simulink model "M_DCMotor_MPC"  (R2019a)
settings: Solver=FixedStepDiscrete  StartTime=0.0  StopTime=18.0  FixedStep=0.0001  RelTol=1e-3
values from neighbouring files (symbols this model uses):
  J = 0.02    [Startfile_M_DCmotor_MPC.m]
  Kemf = 0.1    [Startfile_M_DCmotor_MPC.m]
  Kf = 0.2    [Startfile_M_DCmotor_MPC.m]
  Km = 0.1    [Startfile_M_DCmotor_MPC.m]
  L = 0.5    [Startfile_M_DCmotor_MPC.m]
  Q0_DC_MPC = [0.01 40000 40000 10]    [Startfile_M_DCmotor_MPC.m]
  R = 2    [Startfile_M_DCmotor_MPC.m]
  R0_DC_MPC = 0.01    [Startfile_M_DCmotor_MPC.m]
  SampleTime = 0.0001    [Startfile_M_DCmotor_MPC.m]
undefined symbols (not defined in the file or in its folder): serial
libraries: powerlib x24, instrumentlib x3
settings Model: Creator=simon  LastModifiedBy=simon
settings OptimizationCC: DefaultParameterBehavior=Inlined  EnhancedBackFolding=on  PassReuseOutputArgsAs=Individual arguments  OptimizeBlockOrder=speed  DifferentSizesBufferReuse=on
settings DebuggingCC: ParameterTunabilityLossMsg=error
settings HardwareCC: ProdBitPerPointer=32  ProdBitPerSizeT=32  ProdBitPerPtrDiffT=32  ProdLargestAtomicInteger=Long  ProdLargestAtomicFloat=Double  ProdWordSize=32  ProdHWDeviceType=ARM Compatible->ARM Cortex
settings SFSimCC: MATLABDynamicMemAlloc=off
settings RTWCC: SystemTargetFile=ert.tlc  TemplateMakefile=ert_default_tmf  GenerateReport=on  RTWUseSimCustomCode=on  IncludeHyperlinkInReport=on  LaunchReport=on  GenerateTraceInfo=on  GenerateTraceReport=on  GenerateTraceReportSl=on  GenerateTraceReportSf=on  GenerateTraceReportEml=on  GenerateCodeMetricsReport=on
settings CodeAppCC: ForceParamTrailComments=on  IgnoreCustomStorageClasses=off  OperatorAnnotations=on  SimulinkDataObjDesc=on  SFDataObjDesc=on  InsertBlockDesc=on
settings ERTTargetCC: TargetLangStandard=C99 (ISO)  GenerateSampleERTMain=on  InlinedParameterPlacement=NonHierarchical  ERTCustomFileTemplate=example_file_process.tlc  GlobalDataDefinition=InSeparateSourceFile  GlobalDataReference=InSeparateHeaderFile  ERTFilePackagingFormat=CompactWithDataFile

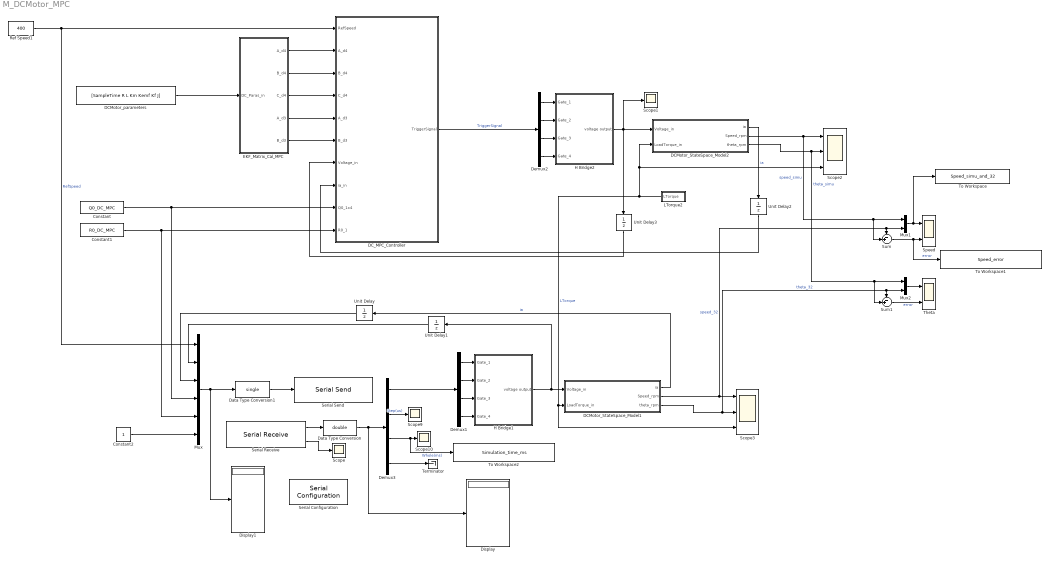
== system M_DCMotor_MPC ==
  Constant : Constant  Value=Q0_DC_MPC
  Constant1 : Constant  Value=R0_DC_MPC
  Constant2 : Constant
  DCMotor_StateSpace_Model1 : Subsystem
  DCMotor_StateSpace_Model2 : Subsystem
  DCMotor_parameters : Constant  Value=[SampleTime R L Km Kemf Kf J]
  DC_MPC_Controller : Subsystem
  Data Type Conversion : DataTypeConversion  OutDataTypeStr=double
  Data Type Conversion1 : DataTypeConversion  OutDataTypeStr=single
  Demux1 : Demux
  Demux2 : Demux
  Demux3 : Demux  Outputs=[4 1 1 3]
  Display : Display
  Display1 : Display
  EKF_Matrix_Cal_MPC : MATLAB Function  TreatAsAtomicUnit=on
  H Bridge1 : Subsystem
  H Bridge2 : Subsystem
  LTorque2 : Subsystem
  Mux : Mux  Inputs=6
  Mux1 : Mux  Inputs=2
  Mux2 : Mux  Inputs=2
  Ref Speed1 : Constant  Value=400
  Scope{,1,9..10} (4 alike) : Scope
  Scope2 : Scope  NumInputPorts=3
  Scope3 : Scope  NumInputPorts=3
  Serial Configuration : instrumentlib/Serial Configuration  Priority=-200000  ComPortMenu=<Please select a port...>  ComPort=/dev/cu.usbmodem141303  ObjConstructor=serial('/dev/cu.usbmodem141303');  BaudRate=921600  DataBits=8  Parity=none  StopBits=1  FlowControl=none  Timeout=10  ByteOrder=LittleEndian
  Serial Receive : instrumentlib/Serial Receive  ComPortMenu=<Please select a port...>  ComPort=/dev/cu.usbmodem141303  ObjConstructor=serial('/dev/cu.usbmodem141303');  Terminator=<none>  DataSize="[1  9]"  DataType=single  EnableBlockingMode=off  ActionDataUnavailable=Output last received value  CustomValue=0  SampleTime=SampleTime
  Serial Send : instrumentlib/Serial Send  ComPortMenu=<Please select a port...>  ComPort=/dev/cu.usbmodem141303  ObjConstructor=serial('/dev/cu.usbmodem141303');  Terminator=<none>  EnableBlockingMode=off
  Speed : Scope  NumInputPorts=2
  Sum : Sum  Inputs=-+|
  Sum1 : Sum  Inputs=-+|
  Terminator : Terminator
  Theta : Scope  NumInputPorts=2
  To Workspace : ToWorkspace  VariableName=Speed_simu_and_32  SampleTime=-1
      settings: Save2DSignal=2-D array (concatenate along first dimension)
  To Workspace1 : ToWorkspace  VariableName=Speed_error  SampleTime=-1
      settings: Save2DSignal=2-D array (concatenate along first dimension)
  To Workspace2 : ToWorkspace  VariableName=Simulation_time_ms  SampleTime=-1
      settings: Save2DSignal=2-D array (concatenate along first dimension)
  Unit Delay{,1..3} (4 alike) : UnitDelay  SampleTime=-1  HasFrameUpgradeWarning=on
  wires:
  DCMotor_parameters/1 -> EKF_Matrix_Cal_MPC/1(DC_Paras_in)
  EKF_Matrix_Cal_MPC/1(A_d4) -> DC_MPC_Controller/2(A_d4)
  EKF_Matrix_Cal_MPC/2(B_d4) -> DC_MPC_Controller/3(B_d4)
  EKF_Matrix_Cal_MPC/3(C_d4) -> DC_MPC_Controller/4(C_d4)
  Constant/1 -> Mux/4, DC_MPC_Controller/9(Q0_1x4)
  Constant1/1 -> Mux/5, DC_MPC_Controller/10(R0_1)
  LTorque2/1(LTorque) -> Scope3/3, DCMotor_StateSpace_Model1/2(LoadTorque_in), DCMotor_StateSpace_Model2/2(LoadTorque_in), Scope2/3  "LTorque"
  Demux2/1 -> H Bridge2/1(Gate_1)
  Demux2/4 -> H Bridge2/4(Gate_4)
  Demux2/3 -> H Bridge2/3(Gate_3)
  H Bridge2/1(voltage output) -> Unit Delay3/1, DCMotor_StateSpace_Model2/1(Voltage_in), Scope1/1
  DC_MPC_Controller/1(TriggerSignal) -> Demux2/1  "TriggerSignal"
  Demux2/2 -> H Bridge2/2(Gate_2)
  DCMotor_StateSpace_Model2/1(ia) -> Unit Delay2/1  "ia"
  DCMotor_StateSpace_Model2/2(Speed_rpm) -> Sum/2, Mux1/1, Scope2/1  "speed_simu"
  DCMotor_StateSpace_Model2/3(theta_rpm) -> Sum1/2, Mux2/1, Scope2/2  "theta_simu"
  Ref Speed1/1 -> Mux/1, DC_MPC_Controller/1(RefSpeed)  "RefSpeed"
  EKF_Matrix_Cal_MPC/4(A_d3) -> DC_MPC_Controller/5(A_d3)
  EKF_Matrix_Cal_MPC/5(B_d3) -> DC_MPC_Controller/6(B_d3)
  Demux3/1 -> Demux1/1
  Demux3/2 -> Scope9/1  "Step(us)"
  Data Type Conversion/1 -> Display/1, Demux3/1
  Demux1/4 -> H Bridge1/4(Gate_4)
  Demux3/3 -> To Workspace2/1, Scope10/1  "Whole(ms)"
  Demux1/2 -> H Bridge1/2(Gate_2)
  Demux1/3 -> H Bridge1/3(Gate_3)
  Mux/1 -> Display1/1, Data Type Conversion1/1
  Demux1/1 -> H Bridge1/1(Gate_1)
  Data Type Conversion1/1 -> Serial Send/1
  Serial Receive/1 -> Data Type Conversion/1
  DCMotor_StateSpace_Model1/3(theta_rpm) -> Mux2/2, Sum1/1, Scope3/2  "theta_32"
  DCMotor_StateSpace_Model1/2(Speed_rpm) -> Sum/1, Mux1/2, Scope3/1  "speed_32"
  H Bridge1/1(voltage output) -> Unit Delay1/1, DCMotor_StateSpace_Model1/1(Voltage_in)
  DCMotor_StateSpace_Model1/1(ia) -> Unit Delay/1  "ia"
  Unit Delay2/1 -> DC_MPC_Controller/8(ia_in)
  Unit Delay3/1 -> DC_MPC_Controller/7(Voltage_in)
  Unit Delay/1 -> Mux/3
  Unit Delay1/1 -> Mux/2
  Demux3/4 -> Terminator/1
  Constant2/1 -> Mux/6
  Mux1/1 -> To Workspace/1, Speed/1
  Sum/1 -> To Workspace1/1, Speed/2  "error"
  Mux2/1 -> Theta/1
  Sum1/1 -> Theta/2  "error"
  Serial Receive/2 -> Scope/1

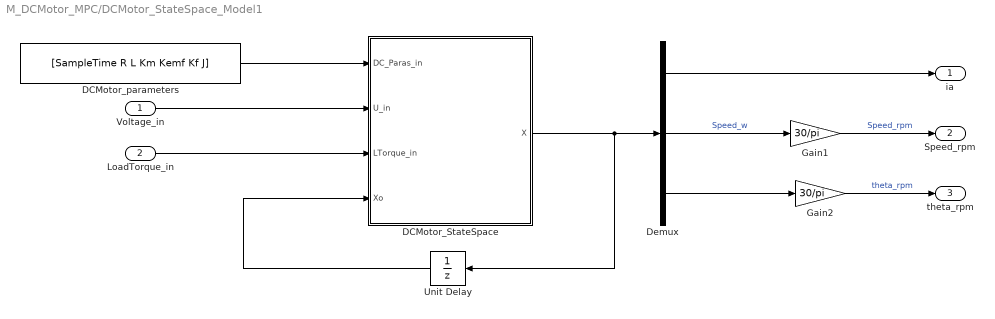
== system M_DCMotor_MPC/DCMotor_StateSpace_Model1 ==
  Voltage_in : Inport
  LoadTorque_in : Inport  Port=2
  DCMotor_StateSpace : MATLAB Function  TreatAsAtomicUnit=on
  DCMotor_parameters : Constant  Value=[SampleTime R L Km Kemf Kf J]
  Demux : Demux  Outputs=3
  Gain1 : Gain  Gain=30/pi
  Gain2 : Gain  Gain=30/pi
  Unit Delay : UnitDelay  SampleTime=-1  HasFrameUpgradeWarning=on
  ia : Outport
  Speed_rpm : Outport  Port=2
  theta_rpm : Outport  Port=3
  wires:
  Gain2/1 -> theta_rpm/1  "theta_rpm"
  Demux/3 -> Gain2/1
  Demux/1 -> ia/1
  Gain1/1 -> Speed_rpm/1  "Speed_rpm"
  Demux/2 -> Gain1/1  "Speed_w"
  DCMotor_StateSpace/1(X) -> Demux/1, Unit Delay/1
  DCMotor_parameters/1 -> DCMotor_StateSpace/1(DC_Paras_in)
  LoadTorque_in/1 -> DCMotor_StateSpace/3(LTorque_in)
  Unit Delay/1 -> DCMotor_StateSpace/4(Xo)
  Voltage_in/1 -> DCMotor_StateSpace/2(U_in)

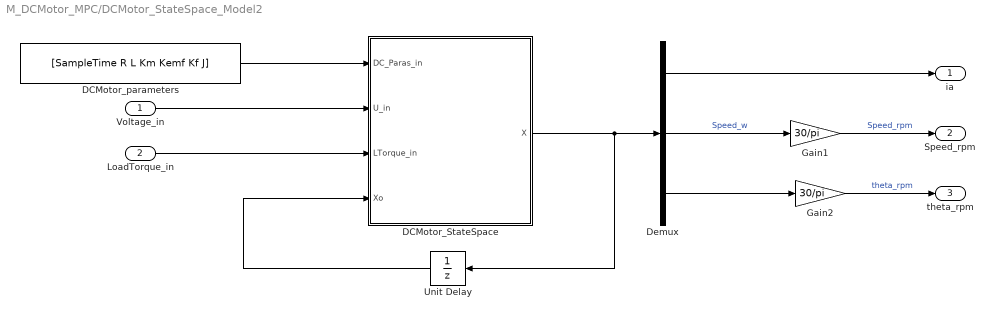
== system M_DCMotor_MPC/DCMotor_StateSpace_Model2 ==
  Voltage_in : Inport
  LoadTorque_in : Inport  Port=2
  DCMotor_StateSpace : MATLAB Function  TreatAsAtomicUnit=on
  DCMotor_parameters : Constant  Value=[SampleTime R L Km Kemf Kf J]
  Demux : Demux  Outputs=3
  Gain1 : Gain  Gain=30/pi
  Gain2 : Gain  Gain=30/pi
  Unit Delay : UnitDelay  SampleTime=-1  HasFrameUpgradeWarning=on
  ia : Outport
  Speed_rpm : Outport  Port=2
  theta_rpm : Outport  Port=3
  wires:
  Voltage_in/1 -> DCMotor_StateSpace/2(U_in)
  Unit Delay/1 -> DCMotor_StateSpace/4(Xo)
  LoadTorque_in/1 -> DCMotor_StateSpace/3(LTorque_in)
  DCMotor_parameters/1 -> DCMotor_StateSpace/1(DC_Paras_in)
  DCMotor_StateSpace/1(X) -> Unit Delay/1, Demux/1
  Demux/2 -> Gain1/1  "Speed_w"
  Gain1/1 -> Speed_rpm/1  "Speed_rpm"
  Demux/1 -> ia/1
  Demux/3 -> Gain2/1
  Gain2/1 -> theta_rpm/1  "theta_rpm"

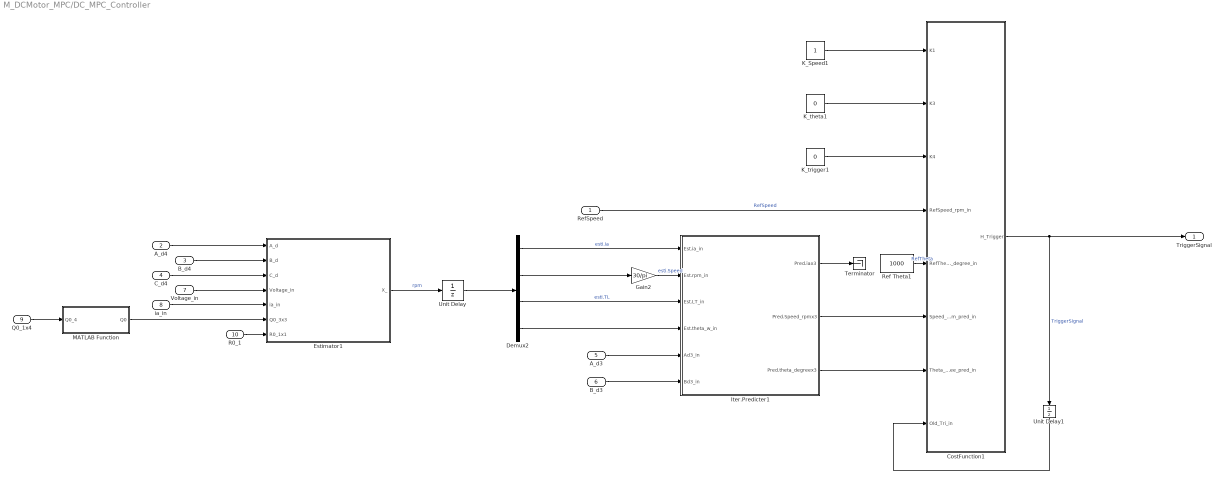
== system M_DCMotor_MPC/DC_MPC_Controller ==
  RefSpeed : Inport
  A_d4 : Inport  Port=2
  B_d4 : Inport  Port=3
  C_d4 : Inport  Port=4
  A_d3 : Inport  Port=5
  B_d3 : Inport  Port=6
  Voltage_in : Inport  Port=7
  ia_in : Inport  Port=8
  Q0_1x4 : Inport  Port=9
  R0_1 : Inport  Port=10
  CostFunction1 : MATLAB Function  TreatAsAtomicUnit=on
  Demux2 : Demux
  Estimator1 : Subsystem
  Gain2 : Gain  Gain=30/pi
  Iter.Predicter1 : Subsystem
  K_Speed1 : Constant
  K_theta1 : Constant  Value=0
  K_trigger1 : Constant  Value=0
  MATLAB Function : MATLAB Function  TreatAsAtomicUnit=on
  Ref Theta1 : Constant  Value=1000
  Terminator : Terminator
  Unit Delay : UnitDelay  SampleTime=-1  HasFrameUpgradeWarning=on
  Unit Delay1 : UnitDelay  SampleTime=-1  HasFrameUpgradeWarning=on
  TriggerSignal : Outport
  wires:
  K_theta1/1 -> CostFunction1/2(K3)
  ia_in/1 -> Estimator1/5(ia_in)
  Demux2/2 -> Gain2/1
  Ref Theta1/1 -> CostFunction1/5(RefTheta_degree_in)  "RefTheta"
  MATLAB Function/1(Q0) -> Estimator1/6(Q0_3x3)
  K_Speed1/1 -> CostFunction1/1(K1)
  R0_1/1 -> Estimator1/7(R0_1x1)
  RefSpeed/1 -> CostFunction1/4(RefSpeed_rpm_in)  "RefSpeed"
  A_d4/1 -> Estimator1/1(A_d)
  Unit Delay1/1 -> CostFunction1/8(Old_Tri_in)
  CostFunction1/1(H_Trigger) -> Unit Delay1/1, TriggerSignal/1  "TriggerSignal"
  Estimator1/1(X_) -> Unit Delay/1  "rpm"
  C_d4/1 -> Estimator1/3(C_d)
  Voltage_in/1 -> Estimator1/4(Voltage_in)
  Q0_1x4/1 -> MATLAB Function/1(Q0_4)
  B_d4/1 -> Estimator1/2(B_d)
  K_trigger1/1 -> CostFunction1/3(K4)
  Gain2/1 -> Iter.Predicter1/2(Est.rpm_in)  "esti.Speed"
  Demux2/3 -> Iter.Predicter1/3(Est.LT_in)  "esti.TL"
  Demux2/1 -> Iter.Predicter1/1(Est.ia_in)  "esti.ia"
  Iter.Predicter1/1(Pred.iax3) -> Terminator/1
  Demux2/4 -> Iter.Predicter1/4(Est.theta_w_in)
  A_d3/1 -> Iter.Predicter1/5(Ad3_in)
  B_d3/1 -> Iter.Predicter1/6(Bd3_in)
  Iter.Predicter1/2(Pred.Speed_rpmx3) -> CostFunction1/6(Speed_rpm_pred_in)
  Iter.Predicter1/3(Pred.theta_degreex3) -> CostFunction1/7(Theta_degree_pred_in)
  Unit Delay/1 -> Demux2/1

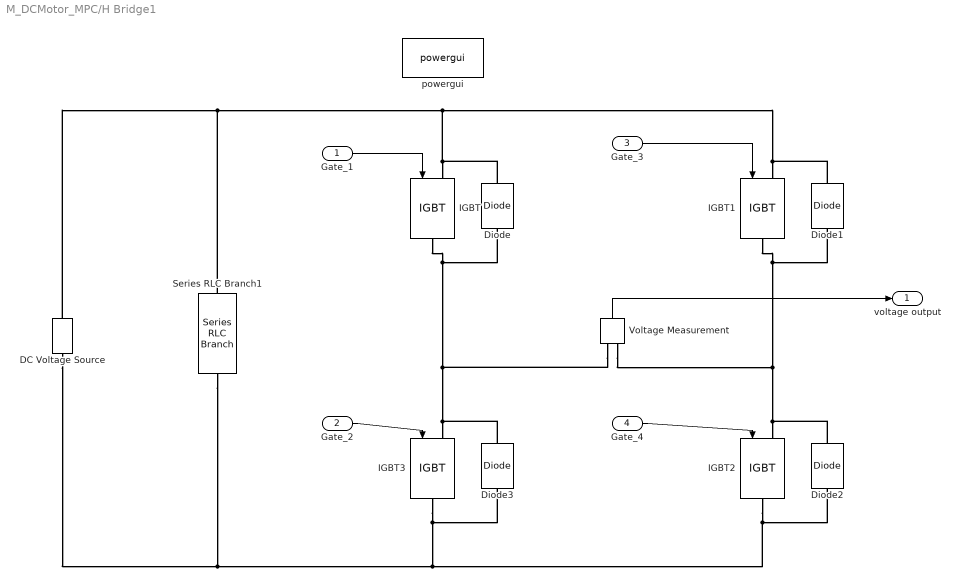
== system M_DCMotor_MPC/H Bridge1 ==
  Gate_1 : Inport
  Gate_2 : Inport  Port=2
  Gate_3 : Inport  Port=3
  Gate_4 : Inport  Port=4
  DC Voltage Source : powerlib/Electrical Sources/DC Voltage Source  Amplitude=400  Measurements=None
      settings: SourceProductName=Simscape Electrical
  Diode{,1..3} (4 alike) : powerlib/Power Electronics/Diode  Ron=0.001  Lon=0  Vf=0.8  IC=0  UseSnubber=0  Rs=500  Cs=250e-9  Measurements=off
      settings: SourceProductName=Simscape Electrical
  IGBT{,1..3} (4 alike) : powerlib/Power Electronics/IGBT  Ron=0.001  Lon=0  Vf=1  Tf=1e-6  Tt=2e-6  IC=0  Rs=1e5  Cs=inf  Measurements=off
      settings: SourceProductName=Simscape Electrical
  Series RLC Branch1 : powerlib/Elements/Series RLC Branch  LConnTagsString=__new0  RConnTagsString=__new0  BranchType=RC  Resistance=0.01  Inductance=1e-3  SetiL0=off  InitialCurrent=0  Capacitance=50e-6  Setx0=off  InitialVoltage=0  Measurements=None
      settings: SourceProductName=Simscape Electrical
  Voltage Measurement : powerlib/Measurements/Voltage Measurement  PhasorSimulation=off  OutputType=Complex  PSBequivalent=0
      settings: SourceProductName=Simscape Electrical
  powergui : powerlib/powergui  Priority=1  SimulationMode=Discrete  SampleTime=0.0001  frequency=60  Iterations=50  frequencyindice=0  Pbase=100e6  ErrMax=1e-4  UnitsV=kV  UnitsW=MW  buscounter=0  FunctionMessages=off  echomessages=off  EnableUseOfTLC=off  CurrentSourceSwitches=off  DisableSnubberDevices=off  DisableRonSwitches=off  DisableVfSwitches=off  DisplayEquations=off  AutomaticDiscreteSolvers=off  SolverType=Tustin/Backward Euler (TBE)  Interpol=off  ExternalGateDelay=off  methode=off  Ts=100  x0status=blocks  SPID=on  SwTol=0  HookPort=off  NonlinearTolerance=0  nMaxIteration=15  ContinueOnMaxIteration=off  RestoreLinks=warning  ResistiveCurrentMeasurement=off  Frange=[0:2:500]  Ylog=off  Xlog=on  ShowGrid=off  save=off  variable=ZData  structure=0  ZoomFFT=off  StartTime=0.0  cycles=1  DisplayStyle=1  fundamental=60  FreqAxis=off  MaxFrequency=1000  frequencyindicesteady=1  RmsSteady=1  display=off
      settings: SourceProductName=Simscape Electrical
  voltage output : Outport
  wires:
  Gate_1/1 -> IGBT/1
  Voltage Measurement/1 -> voltage output/1
  Gate_2/1 -> IGBT3/1
  Gate_3/1 -> IGBT1/1
  Gate_4/1 -> IGBT2/1
  connections:
  IGBT/RConn1 -- Voltage Measurement/LConn1 -- IGBT3/LConn1 -- Diode3/RConn1 -- Diode/LConn1
  Diode/RConn1 -- Series RLC Branch1/LConn1 -- DC Voltage Source/RConn1 -- IGBT1/LConn1 -- Diode1/RConn1 -- IGBT/LConn1
  IGBT1/RConn1 -- Voltage Measurement/LConn2 -- IGBT2/LConn1 -- Diode2/RConn1 -- Diode1/LConn1
  IGBT3/RConn1 -- DC Voltage Source/LConn1 -- Series RLC Branch1/RConn1 -- IGBT2/RConn1 -- Diode2/LConn1 -- Diode3/LConn1

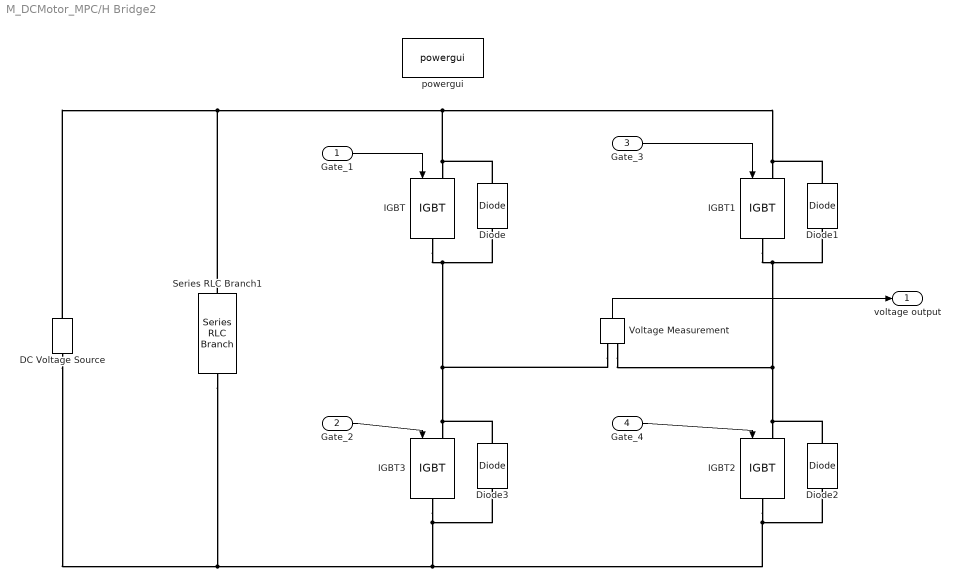
== system M_DCMotor_MPC/H Bridge2 ==
  Gate_1 : Inport
  Gate_2 : Inport  Port=2
  Gate_3 : Inport  Port=3
  Gate_4 : Inport  Port=4
  DC Voltage Source : powerlib/Electrical Sources/DC Voltage Source  Amplitude=400  Measurements=None
      settings: SourceProductName=Simscape Electrical
  Diode{,1..3} (4 alike) : powerlib/Power Electronics/Diode  Ron=0.001  Lon=0  Vf=0.8  IC=0  UseSnubber=0  Rs=500  Cs=250e-9  Measurements=off
      settings: SourceProductName=Simscape Electrical
  IGBT{,1..3} (4 alike) : powerlib/Power Electronics/IGBT  Ron=0.001  Lon=0  Vf=1  Tf=1e-6  Tt=2e-6  IC=0  Rs=1e5  Cs=inf  Measurements=off
      settings: SourceProductName=Simscape Electrical
  Series RLC Branch1 : powerlib/Elements/Series RLC Branch  LConnTagsString=__new0  RConnTagsString=__new0  BranchType=RC  Resistance=0.01  Inductance=1e-3  SetiL0=off  InitialCurrent=0  Capacitance=50e-6  Setx0=off  InitialVoltage=0  Measurements=None
      settings: SourceProductName=Simscape Electrical
  Voltage Measurement : powerlib/Measurements/Voltage Measurement  PhasorSimulation=off  OutputType=Complex  PSBequivalent=0
      settings: SourceProductName=Simscape Electrical
  powergui : powerlib/powergui  Priority=1  SimulationMode=Discrete  SampleTime=0.0001  frequency=60  Iterations=50  frequencyindice=0  Pbase=100e6  ErrMax=1e-4  UnitsV=kV  UnitsW=MW  buscounter=0  FunctionMessages=off  echomessages=off  EnableUseOfTLC=off  CurrentSourceSwitches=off  DisableSnubberDevices=off  DisableRonSwitches=off  DisableVfSwitches=off  DisplayEquations=off  AutomaticDiscreteSolvers=off  SolverType=Tustin/Backward Euler (TBE)  Interpol=off  ExternalGateDelay=off  methode=off  Ts=100  x0status=blocks  SPID=on  SwTol=0  HookPort=off  NonlinearTolerance=0  nMaxIteration=15  ContinueOnMaxIteration=off  RestoreLinks=warning  ResistiveCurrentMeasurement=off  Frange=[0:2:500]  Ylog=off  Xlog=on  ShowGrid=off  save=off  variable=ZData  structure=0  ZoomFFT=off  StartTime=0.0  cycles=1  DisplayStyle=1  fundamental=60  FreqAxis=off  MaxFrequency=1000  frequencyindicesteady=1  RmsSteady=1  display=off
      settings: SourceProductName=Simscape Electrical
  voltage output : Outport
  wires:
  Gate_1/1 -> IGBT/1
  Voltage Measurement/1 -> voltage output/1
  Gate_2/1 -> IGBT3/1
  Gate_3/1 -> IGBT1/1
  Gate_4/1 -> IGBT2/1
  connections:
  IGBT/RConn1 -- Voltage Measurement/LConn1 -- IGBT3/LConn1 -- Diode3/RConn1 -- Diode/LConn1
  Diode/RConn1 -- Series RLC Branch1/LConn1 -- DC Voltage Source/RConn1 -- IGBT1/LConn1 -- Diode1/RConn1 -- IGBT/LConn1
  IGBT1/RConn1 -- Voltage Measurement/LConn2 -- IGBT2/LConn1 -- Diode2/RConn1 -- Diode1/LConn1
  IGBT3/RConn1 -- DC Voltage Source/LConn1 -- Series RLC Branch1/RConn1 -- IGBT2/RConn1 -- Diode2/LConn1 -- Diode3/LConn1

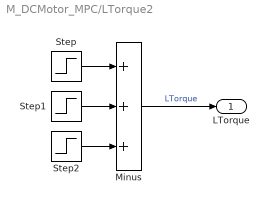
== system M_DCMotor_MPC/LTorque2 ==
  Minus : Sum  Inputs=+++
  Step : Step  Time=4  After=3  SampleTime=0
  Step1 : Step  Time=8  SampleTime=0
  Step2 : Step  Time=12  After=4  SampleTime=0
  LTorque : Outport
  wires:
  Minus/1 -> LTorque/1  "LTorque"
  Step/1 -> Minus/1
  Step1/1 -> Minus/2
  Step2/1 -> Minus/3

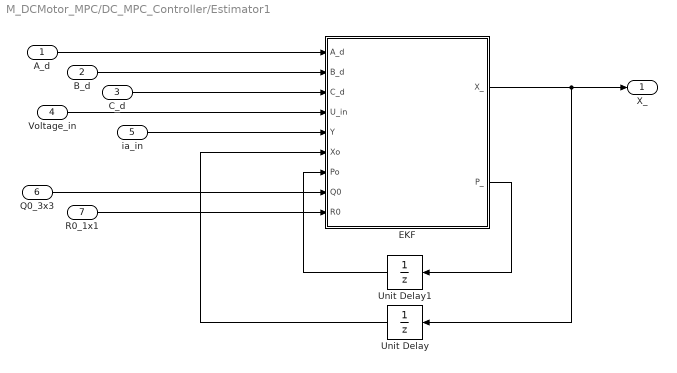
== system M_DCMotor_MPC/DC_MPC_Controller/Estimator1 ==
  A_d : Inport
  B_d : Inport  Port=2
  C_d : Inport  Port=3
  Voltage_in : Inport  Port=4
  ia_in : Inport  Port=5
  Q0_3x3 : Inport  Port=6
  R0_1x1 : Inport  Port=7
  EKF : MATLAB Function  TreatAsAtomicUnit=on
  Unit Delay : UnitDelay  SampleTime=-1  HasFrameUpgradeWarning=on
  Unit Delay1 : UnitDelay  SampleTime=-1  HasFrameUpgradeWarning=on
  X_ : Outport
  wires:
  R0_1x1/1 -> EKF/9(R0)
  Q0_3x3/1 -> EKF/8(Q0)
  Unit Delay1/1 -> EKF/7(Po)
  EKF/2(P_) -> Unit Delay1/1
  EKF/1(X_) -> Unit Delay/1, X_/1
  A_d/1 -> EKF/1(A_d)
  ia_in/1 -> EKF/5(Y)
  Unit Delay/1 -> EKF/6(Xo)
  Voltage_in/1 -> EKF/4(U_in)
  B_d/1 -> EKF/2(B_d)
  C_d/1 -> EKF/3(C_d)

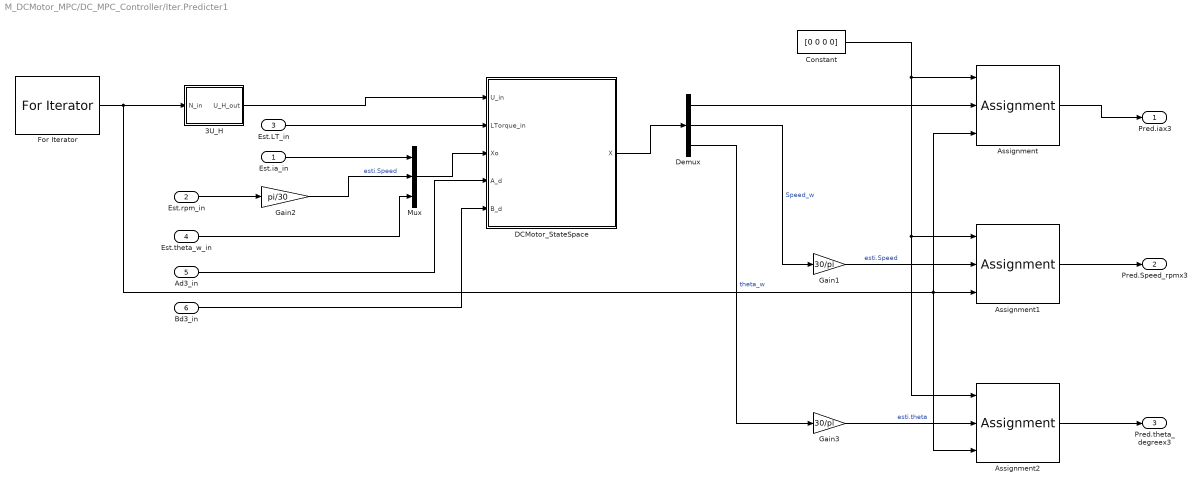
== system M_DCMotor_MPC/DC_MPC_Controller/Iter.Predicter1 ==
  Est.ia_in : Inport
  Est.rpm_in : Inport  Port=2
  Est.LT_in : Inport  Port=3
  Est.theta_w_in : Inport  Port=4
  Ad3_in : Inport  Port=5
  Bd3_in : Inport  Port=6
  3U_H : MATLAB Function  TreatAsAtomicUnit=on
  Assignment : Assignment  DiagnosticForDimensions=Warning  IndexOptions=Index vector (port)  Indices=1  OutputSizes=1
  Assignment1 : Assignment  DiagnosticForDimensions=Warning  IndexOptions=Index vector (port)  Indices=1  OutputSizes=1
  Assignment2 : Assignment  DiagnosticForDimensions=Warning  IndexOptions=Index vector (port)  Indices=1  OutputSizes=1
  Constant : Constant  Value=[0 0 0 0]
  DCMotor_StateSpace : MATLAB Function  TreatAsAtomicUnit=on
  Demux : Demux  Outputs=3
  For Iterator : ForIterator  IterationLimit=4  IterationVariableDataType=int8
  Gain1 : Gain  Gain=30/pi
  Gain2 : Gain  Gain=pi/30
  Gain3 : Gain  Gain=30/pi
  Mux : Mux  Inputs=3
  Pred.iax3 : Outport
  Pred.Speed_rpmx3 : Outport  Port=2
  Pred.theta_degreex3 : Outport  Port=3
  wires:
  DCMotor_StateSpace/1(X) -> Demux/1
  Est.LT_in/1 -> DCMotor_StateSpace/2(LTorque_in)
  3U_H/1(U_H_out) -> DCMotor_StateSpace/1(U_in)
  Demux/2 -> Gain1/1  "Speed_w"
  Demux/1 -> Assignment/2
  For Iterator/1 -> Assignment2/3, Assignment/3, Assignment1/3, 3U_H/1(N_in)
  Mux/1 -> DCMotor_StateSpace/3(Xo)
  Est.ia_in/1 -> Mux/1
  Est.rpm_in/1 -> Gain2/1
  Constant/1 -> Assignment1/1, Assignment2/1, Assignment/1
  Assignment/1 -> Pred.iax3/1
  Assignment1/1 -> Pred.Speed_rpmx3/1
  Gain1/1 -> Assignment1/2  "esti.Speed"
  Gain2/1 -> Mux/2  "esti.Speed"
  Demux/3 -> Gain3/1  "theta_w"
  Est.theta_w_in/1 -> Mux/3
  Assignment2/1 -> Pred.theta_degreex3/1
  Gain3/1 -> Assignment2/2  "esti.theta"
  Ad3_in/1 -> DCMotor_StateSpace/4(A_d)
  Bd3_in/1 -> DCMotor_StateSpace/5(B_d)

== matlab function M_DCMotor_MPC/EKF_Matrix_Cal_MPC ==
  data: DC_Paras_in input; A_d4 output; B_d4 output; C_d4 output; A_d3 output; B_d3 output
function [A_d4,B_d4,C_d4,A_d3,B_d3] = EKF_Matrix_Cal(DC_Paras_in)

SampleTime=DC_Paras_in(1);
R=DC_Paras_in(2);         %Resistor
L=DC_Paras_in(3);       %Inductor
Km=DC_Paras_in(4);      %Torque Constant
Kemf=DC_Paras_in(5);    %Back EMF Voltage Constant
Kf=DC_Paras_in(6);      %Viscous Friction Constant
J=DC_Paras_in(7);      %Inertial Load

%{
    State eqaution:     Xo = A_4x4 * X + B_4x1 * U
    Output equation:    Y = C_1x4 * X + D_1x1 * U
    X = [i_a;w;TL;theta]           armature current; speed(rad/s); load torque
    U = [U_in]       input voltage
    Y = [i_a]
%}

% i_a=Xo(1);
% w=Xo(2);
%U_in=0;

A_4x4=[-R/L -Kemf/L 0 0; Km/J -Kf/J -1/J 0; 0 0 0 0; 0 1 0 0];
B_4x1=[1/L;0;0;0];
C_1x4=[1 0 0 0];
%D_1x1=0;

%Disretization
A_d4 = eye(4) + SampleTime*A_4x4 + (1/2)*SampleTime*SampleTime*A_4x4*A_4x4;
B_d4 = SampleTime*B_4x1+(1/2)*SampleTime*SampleTime*A_4x4*B_4x1;
C_d4 = C_1x4;
%D_d = D_1x1;

%Iterater
A_3x3=[-R/L -Kemf/L 0; Km/J -Kf/J 0; 0 1 0];
B_3x2=[1/L 0; 0 -1/J; 0 0];
%C_1x2=[0 1];

%Disretization
A_d3 = eye(3) + SampleTime*A_3x3 + (1/2)*SampleTime*SampleTime*A_3x3*A_3x3;
B_d3 = SampleTime*B_3x2+(1/2)*SampleTime*SampleTime*A_3x3*B_3x2;

end

== matlab function M_DCMotor_MPC/DC_MPC_Controller/CostFunction1 ==
  data: K1 input; K3 input; K4 input; RefSpeed_rpm_in input; RefTheta_degree_in input; H_Trigger output; Speed_rpm_pred_in input; Theta_degree_pred_in input; Old_Tri_in input size=[1 4]
function H_Trigger  = CostFunction(K1,K3,K4,RefSpeed_rpm_in,RefTheta_degree_in,Speed_rpm_pred_in,Theta_degree_pred_in,Old_Tri_in)

    J_last=10^5;
    Trigger_num=1;
    
    persistent Trigger
    if isempty(Trigger)
        Trigger=[1 0 0 1;0 1 1 0; 1 0 1 0; 0 1 0 1];     
        % H_Trigger=[1 0 0 1];       400V
        % H_Trigger=[0 1 1 0];       -400V
        % H_Trigger=[1 0 1 0];       0V
        % H_Trigger=[0 1 0 1];       0V
    end
    
    for i=1:4
        J=K1*(RefSpeed_rpm_in-Speed_rpm_pred_in(i))^2+...
            K3*(RefTheta_degree_in-Theta_degree_pred_in(i))^2+K4*norm((Trigger(i,:)-Old_Tri_in),1);
        if J<J_last
            J_last=J;
            Trigger_num=i;
        end
    end
    
    H_Trigger=Trigger(Trigger_num,:);
 
end

== matlab function M_DCMotor_MPC/DCMotor_StateSpace_Model1/DCMotor_StateSpace ==
  data: DC_Paras_in input; X output size=[3 1]; U_in input; LTorque_in input; Xo input size=[3 1]
function X = DCMotorStateSpace(DC_Paras_in,U_in,LTorque_in,Xo)

SampleTime=DC_Paras_in(1);
R=DC_Paras_in(2);         %Resistor
L=DC_Paras_in(3);       %Inductor
Km=DC_Paras_in(4);      %Torque Constant
Kemf=DC_Paras_in(5);    %Back EMF Voltage Constant
Kf=DC_Paras_in(6);      %Viscous Friction Constant
J=DC_Paras_in(7);      %Inertial Load

%{
    State eqaution:     Xo = A_3x3 * X + B_3x2 * U
    Output equation:    Y = C_1x2 * X
    X = [i_a;w;θ theta]           armature current; speed(rad/s)
    U = [U_in;Td]       input voltage; Load Torque
    Y = [w] = X(2);
%}

% i_a=Xo(1);
% w=Xo(2);
U=zeros(2,1);
U(1)=U_in;
U(2)=LTorque_in;

A_3x3=[-R/L -Kemf/L 0; Km/J -Kf/J 0; 0 1 0];
B_3x2=[1/L 0; 0 -1/J; 0 0];
%C_1x2=[0 1];

%Disretization
A_d = eye(3) + SampleTime*A_3x3 + (1/2)*SampleTime*SampleTime*A_3x3*A_3x3;
B_d = SampleTime*B_3x2+(1/2)*SampleTime*SampleTime*A_3x3*B_3x2;
%C_d = C_1x2;

%equations
X   = A_d*Xo + B_d*U;
%Y   = C_d*X;

end

== matlab function M_DCMotor_MPC/DC_MPC_Controller/Estimator1/EKF ==
  data: A_d input; B_d input; C_d input; X_ output size=[4 1]; U_in input; Y input; Xo input size=[4 1]; Po input; P_ output; Q0 input; R0 input
function [X_,P_] = DCMotorStateSpace(A_d,B_d,C_d,U_in,Y,Xo,Po,Q0,R0)

% SampleTime=DC_Paras_in(1);
% R=DC_Paras_in(2);         %Resistor
% L=DC_Paras_in(3);       %Inductor
% Km=DC_Paras_in(4);      %Torque Constant
% Kemf=DC_Paras_in(5);    %Back EMF Voltage Constant
% Kf=DC_Paras_in(6);      %Viscous Friction Constant
% J=DC_Paras_in(7);      %Inertial Load

%{
    State eqaution:     Xo = A_3x3 * X + B_3x1 * U
    Output equation:    Y = C_1x3 * X + D_1x1 * U
    X = [i_a;w;TL]           armature current; speed(rad/s); load torque
    U = [U_in]       input voltage
    Y = [i_a]
%}

% i_a=Xo(1);
% w=Xo(2);
%U_in=0;

% A_3x3=[-R/L -Kemf/L 0; Km/J -Kf/J -1/J; 0 0 0];
% B_3x1=[1/L;0;0];
% C_1x3=[1 0 0];
% %D_1x1=0;
% 
% %Disretization
% A_d = eye(3) + SampleTime*A_3x3 + (1/2)*SampleTime*SampleTime*A_3x3*A_3x3;
% B_d = SampleTime*B_3x1+(1/2)*SampleTime*SampleTime*A_3x3*B_3x1;
% C_d = C_1x3;
% %D_d = D_1x1;

%pridiction
X_star  = A_d*Xo + B_d*U_in;
Y_star  = C_d*X_star;

% Initialization ...
% X0      = [0 0 0 0 0 0]';
% Q0      = diag([1 1 1 1 1 1]);
% R0      = diag([1 1]);
% P_      = ones(6,6);

% Gradient Matrcies ...
% F_3x3   = A_d;
% H_1x3   = C_d;

% Covariance Matercies ...
% P_star  = F_3x3*Po*F_3x3' + Q0;
% K_      = P_star*H_1x3'*(H_1x3*P_star*H_1x3' + R0)^-1;
% P_      = P_star - K_*H_1x3*P_star;
% X_      = X_star + K_*(Y - Y_star);

P_star  = A_d*Po*A_d' + Q0;
K_      = P_star*C_d'*(C_d*P_star*C_d' + R0)^-1;
P_      = P_star - K_*C_d*P_star;
X_      = X_star + K_*(Y - Y_star);

end

== matlab function M_DCMotor_MPC/DC_MPC_Controller/MATLAB Function ==
  data: Q0_4 input; Q0 output
function Q0 = Q0_extend(Q0_4)

Q0=zeros(4);
Q0(1,1)=Q0_4(1);
Q0(2,2)=Q0_4(2);
Q0(3,3)=Q0_4(3);
Q0(4,4)=Q0_4(4);

end

== matlab function M_DCMotor_MPC/DC_MPC_Controller/Iter.Predicter1/3U_H ==
  data: N_in input; U_H_out output
function U_H_out = U_H(N_in)

switch N_in
    case 1
        U_H_out=400;
    case 2
        U_H_out=-400;
    case 3
        U_H_out=0;
    otherwise
        U_H_out=0;
end

end

== matlab function M_DCMotor_MPC/DC_MPC_Controller/Iter.Predicter1/DCMotor_StateSpace ==
  data: U_in input; LTorque_in input; Xo input size=[3 1]; A_d input; X output size=[3 1]; B_d input
function X = DCMotorStateSpace(U_in,LTorque_in,Xo,A_d,B_d)

% SampleTime=DC_Paras_in(1);
% R=DC_Paras_in(2);         %Resistor
% L=DC_Paras_in(3);       %Inductor
% Km=DC_Paras_in(4);      %Torque Constant
% Kemf=DC_Paras_in(5);    %Back EMF Voltage Constant
% Kf=DC_Paras_in(6);      %Viscous Friction Constant
% J=DC_Paras_in(7);      %Inertial Load

%{
    State eqaution:     Xo = A_3x3 * X + B_3x2 * U
    Output equation:    Y = C_1x2 * X
    X = [i_a;w;θ theta]           armature current; speed(rad/s)
    U = [U_in;Td]       input voltage; Load Torque
    Y = [w] = X(2);
%}

% i_a=Xo(1);
% w=Xo(2);
U=zeros(2,1);
U(1)=U_in;
U(2)=LTorque_in;

% A_3x3=[-R/L -Kemf/L 0; Km/J -Kf/J 0; 0 1 0];
% B_3x2=[1/L 0; 0 -1/J; 0 0];
% %C_1x2=[0 1];
% 
% %Disretization
% A_d = eye(3) + SampleTime*A_3x3 + (1/2)*SampleTime*SampleTime*A_3x3*A_3x3;
% B_d = SampleTime*B_3x2+(1/2)*SampleTime*SampleTime*A_3x3*B_3x2;
% %C_d = C_1x2;

%equations
X   = A_d*Xo + B_d*U;
%Y   = C_d*X;

end

== matlab function M_DCMotor_MPC/DCMotor_StateSpace_Model2/DCMotor_StateSpace ==
  data: DC_Paras_in input; X output size=[3 1]; U_in input; LTorque_in input; Xo input size=[3 1]
function X = DCMotorStateSpace(DC_Paras_in,U_in,LTorque_in,Xo)

SampleTime=DC_Paras_in(1);
R=DC_Paras_in(2);         %Resistor
L=DC_Paras_in(3);       %Inductor
Km=DC_Paras_in(4);      %Torque Constant
Kemf=DC_Paras_in(5);    %Back EMF Voltage Constant
Kf=DC_Paras_in(6);      %Viscous Friction Constant
J=DC_Paras_in(7);      %Inertial Load

%{
    State eqaution:     Xo = A_3x3 * X + B_3x2 * U
    Output equation:    Y = C_1x2 * X
    X = [i_a;w;θ theta]           armature current; speed(rad/s)
    U = [U_in;Td]       input voltage; Load Torque
    Y = [w] = X(2);
%}

% i_a=Xo(1);
% w=Xo(2);
U=zeros(2,1);
U(1)=U_in;
U(2)=LTorque_in;

A_3x3=[-R/L -Kemf/L 0; Km/J -Kf/J 0; 0 1 0];
B_3x2=[1/L 0; 0 -1/J; 0 0];
%C_1x2=[0 1];

%Disretization
A_d = eye(3) + SampleTime*A_3x3 + (1/2)*SampleTime*SampleTime*A_3x3*A_3x3;
B_d = SampleTime*B_3x2+(1/2)*SampleTime*SampleTime*A_3x3*B_3x2;
%C_d = C_1x2;

%equations
X   = A_d*Xo + B_d*U;
%Y   = C_d*X;

end
